simulink model "MultiportSwitch_TestGen5"  (R2017b)
settings: Solver=FixedStepDiscrete  StartTime=0.0  StopTime=10.0  RelTol=1e-3
settings Model: Creator=ktrinh  LastModifiedBy=ktrinh
settings DebuggingCC: ParameterOverflowMsg=none

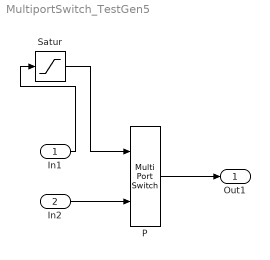
== system MultiportSwitch_TestGen5 ==
  In1 : Inport  OutMin=0  OutMax=1
  In2 : Inport  Port=2  PortDimensions=[1,5]
  P : MultiPortSwitch  DataPortOrder=Zero-based contiguous  Inputs=1  DataPortForDefault=Additional data port
  Satur : Saturate  UpperLimit=1  LowerLimit=0
  Out1 : Outport
  wires:
  In2/1 -> P/2
  P/1 -> Out1/1
  In1/1 -> Satur/1
  Satur/1 -> P/1
